simulink model "Simu_LQRZ"  (R2018a)
settings: Solver=VariableStepAuto  StartTime=0.0  StopTime=1000  RelTol=1e-3
values from neighbouring files (symbols this model uses):
  A = [  0  1  0  0 ... (first row only)    [Dados.m]    (also in Function_ARE.m = [A, zeros(4,2); SDRE.m; areklmn_reactor.m = [A, zeros(4,2); fd0.m = [A, zeros(4,2))
  B = [ 0  0 ... (first row only)    [Dados.m]    (also in Dados_correct.m; Function_ARE.m = [B; SDRE.m; areklmn_reactor.m = [B)
  C = [1 0 0 0 ... (first row only)    [Dados.m]    (also in Dados_correct.m; Function_ARE.m = D; teste.m = D)
  K1 = Kpi(:,1:4)    [Dados.m]    (also in Dados_correct.m = Kpi90(:,1:4); Function_ARE.m = K(:,1:4); teste.m = K(:,1:4))
  K2 = Kpi(:,5:6)    [Dados.m]    (also in Dados_correct.m = Kpi90(:,5:6); Function_ARE.m = K(:,5:6); teste.m = K(:,5:6))
settings Model: Creator=stayn  LastModifiedBy=stayn

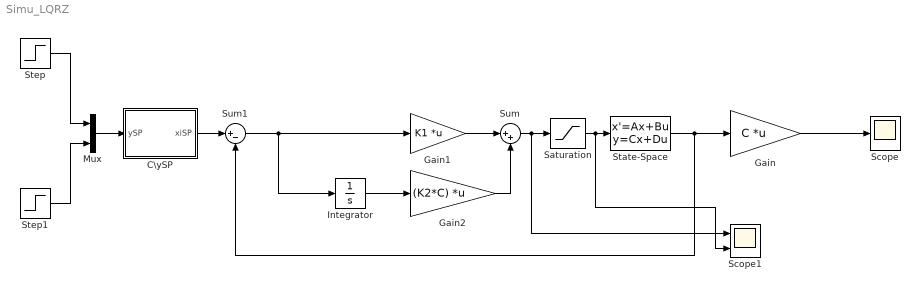
== system Simu_LQRZ ==
  C\ySP : MATLAB Function  TreatAsAtomicUnit=on
  Gain : Gain  Gain=C  Multiplication=Matrix(K*u) (u vector)
  Gain1 : Gain  Gain=K1  Multiplication=Matrix(K*u) (u vector)
  Gain2 : Gain  Gain=(K2*C)  Multiplication=Matrix(K*u) (u vector)
  Integrator : Integrator
  Mux : Mux  Inputs=2
  Saturation : Saturate  UpperLimit=11  LowerLimit=-5
  Scope : Scope
  Scope1 : Scope  NumInputPorts=2
  State-Space : StateSpace  A=A  B=B  C=eye(4)  D=zeros(4,2)  InitialCondition=[0 0 0 0]
  Step : Step  SampleTime=0
  Step1 : Step  After=0  SampleTime=0
  Sum : Sum  Inputs=|++
  Sum1 : Sum  Inputs=|+-
  wires:
  State-Space/1 -> Sum1/2, Gain/1
  Gain/1 -> Scope/1
  Gain1/1 -> Sum/1
  Sum/1 -> Saturation/1, Scope1/1
  Gain2/1 -> Sum/2
  Integrator/1 -> Gain2/1
  Step1/1 -> Mux/2
  Step/1 -> Mux/1
  Mux/1 -> C\ySP/1(ySP)
  Sum1/1 -> Integrator/1, Gain1/1
  C\ySP/1(xiSP) -> Sum1/1
  Saturation/1 -> Scope1/2, State-Space/1

== matlab function Simu_LQRZ/C\ySP ==
  data: ySP input; xiSP output
function xiSP = fcn(ySP)

C = [1 0 0 0;
     0 0 1 0];

xiSP = C\ySP;
